simulink model "DroneControlSimulink"  (R2026a)
settings: Solver=VariableStepAuto  StopTime=25
values from neighbouring files (symbols this model uses):
  b = C_T*rho_A*D^4    (= 7.687659375e-05)    [drone_params.m]
  d = C_p*rho_A*D^5    (= 4.71742734375e-06)    [drone_params.m]
  g = 9.81    [drone_params.m]
  J_r = 15e-6    (= 1.5e-05)    [drone_params.m]
  l = 0.2    [drone_params.m]
  m = 0.568    [drone_params.m]
undefined symbols (not defined in the file or in its folder): J_xx, J_yy, J_zz, K_dx, K_dy, K_dz, K_LQR, traj_points, traj_times, w_max, w_min, X0
libraries: cstblocks_lti x4
settings Model: Creator=andit  LastModifiedBy=andreasthoeni

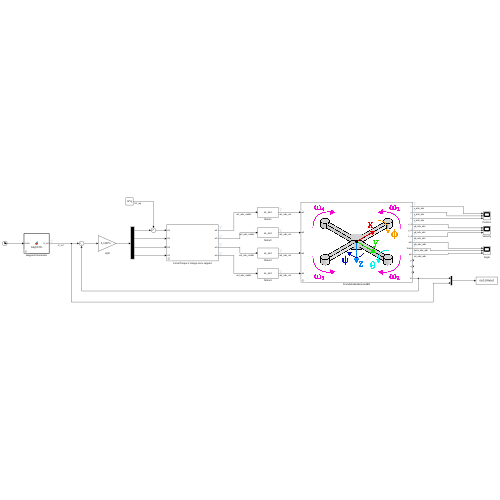
[thumbnail: Simulink's stored preview of the top-level diagram]
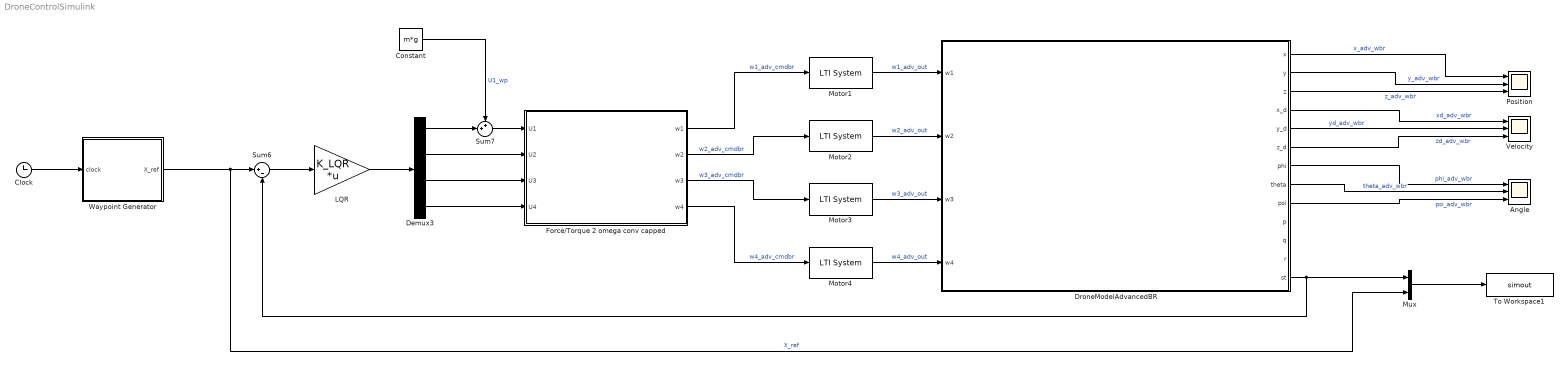
== system DroneControlSimulink ==
  Angle : Scope  NumInputPorts=3
      settings: ActiveDisplayYMinimum=-1  ActiveDisplayYMaximum=1  DataLoggingVariableName=ScopeData6
  Clock : Clock
  Constant : Constant  Value=m*g
  Demux3 : Demux
  DroneModelAdvancedBR : Subsystem  mask{m=m, g=g, l=l, I_xx=J_xx, I_yy=J_yy, I_zz=J_zz, J_r=J_r, b=b, d=d, K_dx=K_dx, K_dy=K_dy, K_dz=K_dz, X0=X0}
      mask prompts: m "mass"; l "length of rotor"; J_r "Motor Inertia J_r"; b "Thrust factor b"; d "Drag factor d"; K_dx "Drag coeff. drone x"; K_dy "Drag coeff. drone y"; K_dz "Drag coeff. drone z"; X0 "Initial conditions"
      mask DialogControl THETA Prompt: Principal Moments of Inertia
      mask DialogControl PROPELLER Prompt: Propeller Coefficients
      mask DialogControl dronedrag Prompt: Drone Drag Coefficients
      mask Display: image('drone_v2.png', [20,10,20,10,100,100]);
  Force/Torque 2 omega conv capped : Subsystem  mask{b=b, d=d, w_max=w_max, w_min=w_min}
      mask prompts: b "Thrust factor b"; d "Drag factor d"; w_max "Maximum"; w_min "Minimum"
      mask DialogControl PROPELLER Prompt: Propeller Coefficients
      mask DialogControl MOTORLIMITS Prompt: Angular velocity limits
  LQR : Gain  Gain=K_LQR  Multiplication=Matrix(K*u)
  Motor{1..4} (4 alike) : cstblocks_lti/LTI System  sys=ss_mot  IC=[]  PadeOrder=0
      settings: LibrarySourceBlock=cstblocks/LTI System
  Mux : Mux  Inputs=2
  Position : Scope  NumInputPorts=3
      settings: ActiveDisplayYMinimum=-6.9992385962365713  ActiveDisplayYMaximum=6.2191487423693133  DataLoggingVariableName=ScopeData4
  Sum6 : Sum  Inputs=|+-
  Sum7 : Sum  Inputs=++|
  To Workspace1 : ToWorkspace  VariableName=simout  SaveFormat=Timeseries  SampleTime=-1
  Velocity : Scope  NumInputPorts=3
      settings: ActiveDisplayYMinimum=-0.125  ActiveDisplayYMaximum=1.125  DataLoggingVariableName=ScopeData5
  Waypoint Generator : MATLAB Function  TreatAsAtomicUnit=on  mask{traj_times=traj_times, traj_points=traj_points}
      mask prompts: traj_times "Waypoint Time Points"; traj_points "Waypoints"
  wires:
  DroneModelAdvancedBR/4(x_d) -> Velocity/1  "xd_adv_wbr"
  DroneModelAdvancedBR/2(y) -> Position/2  "y_adv_wbr"
  Constant/1 -> Sum7/1  "U1_wp"
  DroneModelAdvancedBR/5(y_d) -> Velocity/2  "yd_adv_wbr"
  DroneModelAdvancedBR/7(phi) -> Angle/1  "phi_adv_wbr"
  Force/Torque 2 omega conv capped/4(w4) -> Motor4/1  "w4_adv_cmdbr"
  DroneModelAdvancedBR/8(theta) -> Angle/2  "theta_adv_wbr"
  DroneModelAdvancedBR/13(st) -> Mux/1, Sum6/2
  Force/Torque 2 omega conv capped/3(w3) -> Motor3/1  "w3_adv_cmdbr"
  DroneModelAdvancedBR/9(psi) -> Angle/3  "psi_adv_wbr"
  Demux3/3 -> Force/Torque 2 omega conv capped/3(U3)
  Waypoint Generator/1(X_ref) -> Mux/2, Sum6/1  "X_ref"
  Mux/1 -> To Workspace1/1
  Sum7/1 -> Force/Torque 2 omega conv capped/1(U1)
  Demux3/1 -> Sum7/2
  DroneModelAdvancedBR/6(z_d) -> Velocity/3  "zd_adv_wbr"
  Force/Torque 2 omega conv capped/2(w2) -> Motor2/1  "w2_adv_cmdbr"
  Sum6/1 -> LQR/1
  DroneModelAdvancedBR/3(z) -> Position/3  "z_adv_wbr"
  Demux3/4 -> Force/Torque 2 omega conv capped/4(U4)
  Motor4/1 -> DroneModelAdvancedBR/4(w4)  "w4_adv_out"
  Demux3/2 -> Force/Torque 2 omega conv capped/2(U2)
  DroneModelAdvancedBR/1(x) -> Position/1  "x_adv_wbr"
  Motor1/1 -> DroneModelAdvancedBR/1(w1)  "w1_adv_out"
  Motor2/1 -> DroneModelAdvancedBR/2(w2)  "w2_adv_out"
  Force/Torque 2 omega conv capped/1(w1) -> Motor1/1  "w1_adv_cmdbr"
  Clock/1 -> Waypoint Generator/1(clock)
  LQR/1 -> Demux3/1
  Motor3/1 -> DroneModelAdvancedBR/3(w3)  "w3_adv_out"

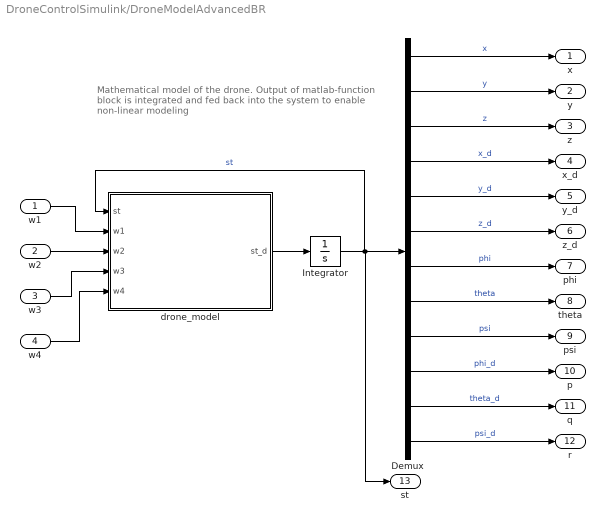
== system DroneControlSimulink/DroneModelAdvancedBR ==
  note: Mathematical model of the drone.
      | Output of matlab-function block is integrated and fed back
      | into the system to enable non-linear modeling
  w1 : Inport
  w2 : Inport  Port=2
  w3 : Inport  Port=3
  w4 : Inport  Port=4
  Demux : Demux  Outputs=12
  Integrator : Integrator  InitialCondition=X0
  drone_model : MATLAB Function  TreatAsAtomicUnit=on
  x : Outport
  y : Outport  Port=2
  z : Outport  Port=3
  x_d : Outport  Port=4
  y_d : Outport  Port=5
  z_d : Outport  Port=6
  phi : Outport  Port=7
  theta : Outport  Port=8
  psi : Outport  Port=9
  p : Outport  Port=10
  q : Outport  Port=11
  r : Outport  Port=12
  st : Outport  Port=13
  wires:
  w2/1 -> drone_model/3(w2)
  w4/1 -> drone_model/5(w4)
  Demux/2 -> y/1  "y"
  Demux/1 -> x/1  "x"
  w1/1 -> drone_model/2(w1)
  w3/1 -> drone_model/4(w3)
  drone_model/1(st_d) -> Integrator/1
  Demux/11 -> q/1  "theta_d"
  Demux/7 -> phi/1  "phi"
  Demux/3 -> z/1  "z"
  Integrator/1 -> Demux/1, st/1, drone_model/1(st)  "st"
  Demux/12 -> r/1  "psi_d"
  Demux/8 -> theta/1  "theta"
  Demux/4 -> x_d/1  "x_d"
  Demux/9 -> psi/1  "psi"
  Demux/5 -> y_d/1  "y_d"
  Demux/10 -> p/1  "phi_d"
  Demux/6 -> z_d/1  "z_d"

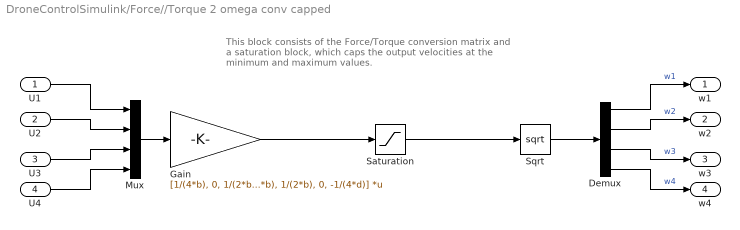
== system DroneControlSimulink/Force//Torque 2 omega conv capped ==
  note: This block  consists of the Force/Torque conversion matrix
      | and a saturation block, which caps the output velocities
      | at the minimum and maximum values.
  U1 : Inport
  U2 : Inport  Port=2
  U3 : Inport  Port=3
  U4 : Inport  Port=4
  Demux : Demux
  Gain : Gain  Gain=|  Multiplication=Matrix(K*u) (u vector)
      | [1/(4*b), 0, 1/(2*b),  1/(4*d); 1/(4*b), -1/(2*b), 0, -1/(4*d);
      | 1/(4*b), 0, -1/(2*b), 1/(4*d);
      | 1/(4*b), 1/(2*b), 0, -1/(4*d)]
  Mux : Mux
  Saturation : Saturate  UpperLimit=w_max^2  LowerLimit=w_min^2
  Sqrt : Sqrt  OutputSignalType=real
  w1 : Outport
  w2 : Outport  Port=2
  w3 : Outport  Port=3
  w4 : Outport  Port=4
  wires:
  Mux/1 -> Gain/1
  Sqrt/1 -> Demux/1
  U1/1 -> Mux/1
  U2/1 -> Mux/2
  Demux/4 -> w4/1  "w4"
  Demux/1 -> w1/1  "w1"
  U4/1 -> Mux/4
  Demux/3 -> w3/1  "w3"
  Demux/2 -> w2/1  "w2"
  U3/1 -> Mux/3
  Gain/1 -> Saturation/1
  Saturation/1 -> Sqrt/1

== matlab function DroneControlSimulink/Waypoint Generator ==
  data: clock input; X_ref output; traj_points parameter; traj_times parameter
function X_ref = waypoints(clock, traj_points, traj_times)

    X_ref = traj_points(1, :);

    for i = 1:length(traj_times)
        if clock >= traj_times(i)
            X_ref = traj_points(i, :);
        end
    end
    X_ref = X_ref';
end

== matlab function DroneControlSimulink/DroneModelAdvancedBR/drone_model ==
  data: st input; st_d output; w1 input; w2 input; w3 input; w4 input; m parameter; g parameter; l parameter; I_xx parameter; I_yy parameter; I_zz parameter; J_r parameter; b parameter; d parameter; K_dx parameter; K_dy parameter; K_dz parameter
function st_d = drone_model(st, w1, w2, w3, w4, m, g, l, I_xx, I_yy, I_zz, J_r, b, d, K_dx, K_dy, K_dz)

% st = [x, y, z, x_d, y_d, z_d, phi, theta, psi, p, q, r]

% lin v and euler angles
x_d = st(4); y_d = st(5); z_d = st(6);
phi = st(7); theta = st(8); psi = st(9);

% body rates
p = st(10); q = st(11); r = st(12);

% motor effects
Omega = w1 - w2 + w3 - w4;
FT_b = b * (w1^2 + w2^2 + w3^2 + w4^2);

% translational
x_dd = (1/m) * (-(cos(phi)*cos(psi)*sin(theta) + sin(phi)*sin(psi))*FT_b - K_dx*x_d);
y_dd = (1/m) * (-(cos(phi)*sin(psi)*sin(theta) - cos(psi)*sin(phi))*FT_b - K_dy*y_d);
z_dd = (1/m) * (-(cos(phi)*cos(theta))*FT_b - K_dz*z_d) + g;

% angular acc in body frame
p_dot = (1/I_xx) * ((I_yy - I_zz)*q*r - J_r*q*Omega + l*b*(w4^2 - w2^2));
q_dot = (1/I_yy) * ((I_zz - I_xx)*p*r + J_r*p*Omega + l*b*(w1^2 - w3^2));
r_dot = (1/I_zz) * ((I_xx - I_yy)*p*q + d*(w1^2 - w2^2 + w3^2 - w4^2));

% body rates 2 euler rates
phi_d   = p + sin(phi)*tan(theta)*q + cos(phi)*tan(theta)*r;
theta_d = cos(phi)*q - sin(phi)*r;
psi_d   = (sin(phi)/cos(theta))*q + (cos(phi)/cos(theta))*r; 

st_d = [x_d;
        y_d;
        z_d;
        x_dd;
        y_dd;
        z_dd;
        phi_d;
        theta_d;
        psi_d;
        p_dot;
        q_dot;
        r_dot];
end
